simulink model "PC_Quadcopter_Simulation_Lyapnov_Hamilton"  (R2015b)
settings: Solver=FixedStepAuto  StartTime=0.0  StopTime=10  FixedStep=0.02  RelTol=1e-3
values from neighbouring files (symbols this model uses):
  IC = block.DialogPrm(2).Data    [QuadHamiSFunctionArticle.m]    (also in initialData.mat = )
  quadModel =     [initialData.mat]
undefined symbols (not defined in the file): K10, K11, K12, K7, K8, K9
settings Model: Creator=HKJ  LastModifiedBy=HL

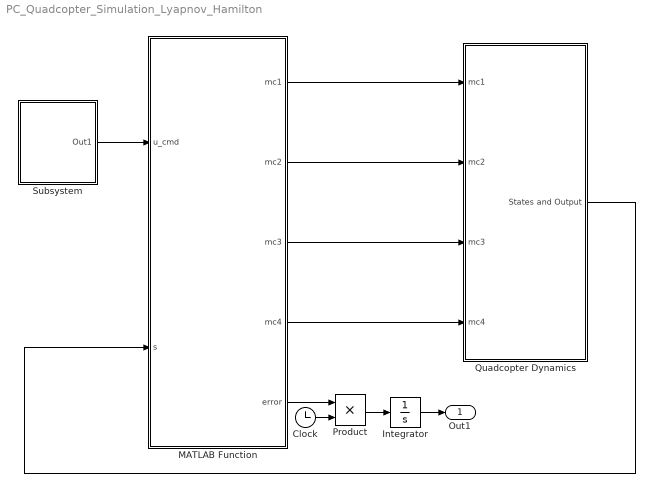
== system PC_Quadcopter_Simulation_Lyapnov_Hamilton ==
  Clock : Clock
  Integrator : Integrator
  MATLAB Function : MATLAB Function  TreatAsAtomicUnit=on  mask{k1=15, k2=8, k3=15, k4=8, k5=2.5, k6=2.5, k7=K7, k8=K8, k9=K9, k10=K10, k11=K11, k12=K12}
  Product : Product
  Quadcopter Dynamics : Subsystem
  Subsystem : Subsystem
  Out1 : Outport
  wires:
  MATLAB Function/1(mc1) -> Quadcopter Dynamics/1(mc1)
  MATLAB Function/2(mc2) -> Quadcopter Dynamics/2(mc2)
  MATLAB Function/3(mc3) -> Quadcopter Dynamics/3(mc3)
  MATLAB Function/4(mc4) -> Quadcopter Dynamics/4(mc4)
  Subsystem/1(Out1) -> MATLAB Function/1(u_cmd)
  Quadcopter Dynamics/1(States and Output) -> MATLAB Function/2(s)
  MATLAB Function/5(error) -> Product/1
  Clock/1 -> Product/2
  Product/1 -> Integrator/1
  Integrator/1 -> Out1/1

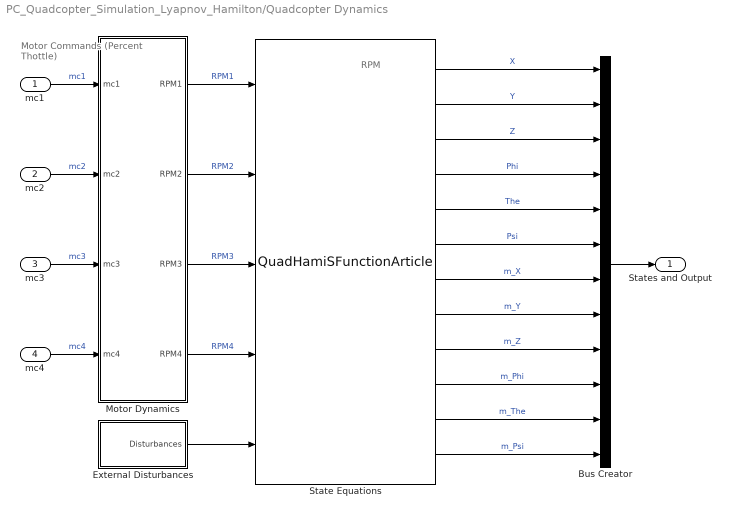
== system PC_Quadcopter_Simulation_Lyapnov_Hamilton/Quadcopter Dynamics ==
  note: Motor Commands
      | (Percent Thottle)
  note: RPM
  mc1 : Inport
  mc2 : Inport  Port=2
  mc3 : Inport  Port=3
  mc4 : Inport  Port=4
  Bus Creator : BusCreator  Inputs='X','Y','Z','Phi','The','Psi','m_X','m_Y','m_Z','m_Phi','m_The','m_Psi'
  External Disturbances : Subsystem
  Motor Dynamics : Subsystem
  State Equations : M-S-Function  FunctionName=QuadHamiSFunctionArticle  Parameters=quadModel,IC
      mask Display:
      | port_label('input', 1, 'RPM1')
      | port_label('input', 2, 'RPM2')
      | port_label('input', 3, 'RPM3')
      | port_label('input', 4, 'RPM4')
      | port_label('input', 5, 'Disturbances')
      | port_label('output', 1, 'X')
      | port_label('output', 2, 'Y')
      | port_label('output', 3, 'Z')
      | port_label('output', 4, 'Phi')
      | port_label('output', 5, 'The')
      | port_label('output', 6, 'Psi')
      | port_label('output', 7, 'm_X')
      | port_label('output', 8, 'm_Y')
      | port_label('output', 9, 'm_Z')
      | port_label('output', 10, 'm_Phi')
      | port_label('output', 11, 'm_The')
      | port_label('output', 12, 'm_Psi')
  States and Output : Outport
  wires:
  mc1/1 -> Motor Dynamics/1(mc1)  "mc1"
  mc2/1 -> Motor Dynamics/2(mc2)  "mc2"
  mc3/1 -> Motor Dynamics/3(mc3)  "mc3"
  mc4/1 -> Motor Dynamics/4(mc4)  "mc4"
  State Equations/1 -> Bus Creator/1  "X"
  State Equations/2 -> Bus Creator/2  "Y"
  State Equations/3 -> Bus Creator/3  "Z"
  State Equations/4 -> Bus Creator/4  "Phi"
  State Equations/5 -> Bus Creator/5  "The"
  State Equations/6 -> Bus Creator/6  "Psi"
  State Equations/7 -> Bus Creator/7  "m_X"
  State Equations/8 -> Bus Creator/8  "m_Y"
  State Equations/9 -> Bus Creator/9  "m_Z"
  State Equations/10 -> Bus Creator/10  "m_Phi"
  State Equations/11 -> Bus Creator/11  "m_The"
  State Equations/12 -> Bus Creator/12  "m_Psi"
  Bus Creator/1 -> States and Output/1
  Motor Dynamics/1(RPM1) -> State Equations/1  "RPM1"
  Motor Dynamics/2(RPM2) -> State Equations/2  "RPM2"
  Motor Dynamics/3(RPM3) -> State Equations/3  "RPM3"
  Motor Dynamics/4(RPM4) -> State Equations/4  "RPM4"
  External Disturbances/1("Disturbances ") -> State Equations/5

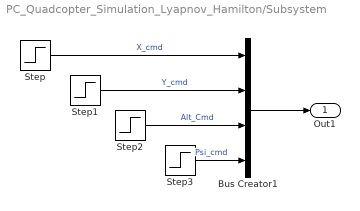
== system PC_Quadcopter_Simulation_Lyapnov_Hamilton/Subsystem ==
  Bus Creator1 : BusCreator  Inputs=4
  Step : Step  Time=0  SampleTime=0
  Step1 : Step  Time=0  SampleTime=0
  Step2 : Step  Time=0  After=-1  SampleTime=0
  Step3 : Step  Time=0  After=0  SampleTime=0
  Out1 : Outport
  wires:
  Step3/1 -> Bus Creator1/4  "Psi_cmd"
  Step2/1 -> Bus Creator1/3  "Alt_Cmd"
  Step/1 -> Bus Creator1/1  "X_cmd"
  Step1/1 -> Bus Creator1/2  "Y_cmd"
  Bus Creator1/1 -> Out1/1

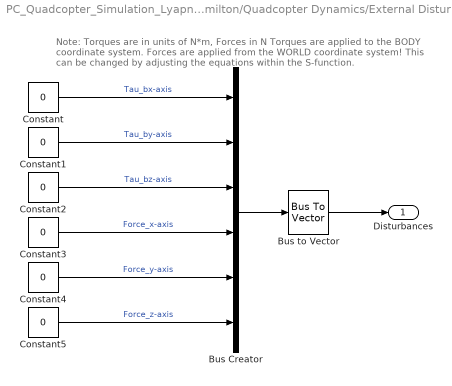
== system PC_Quadcopter_Simulation_Lyapnov_Hamilton/Quadcopter Dynamics/External Disturbances ==
  note: Note: Torques are in units of N*m, Forces in N
      | Torques are applied to the BODY coordinate system.
      | Forces are applied from the WORLD coordinate system!
      | This can be changed by adjusting the equations within the S-function.
  Bus Creator : BusCreator  Inputs=6
  Bus to Vector : BusToVector
  Constant{,1..5} (6 alike) : Constant  Value=0
  "Disturbances " : Outport
  wires:
  Bus to Vector/1 -> "Disturbances "/1
  Bus Creator/1 -> Bus to Vector/1
  Constant/1 -> Bus Creator/1  "Tau_bx-axis"
  Constant1/1 -> Bus Creator/2  "Tau_by-axis"
  Constant2/1 -> Bus Creator/3  "Tau_bz-axis"
  Constant3/1 -> Bus Creator/4  "Force_x-axis"
  Constant4/1 -> Bus Creator/5  "Force_y-axis"
  Constant5/1 -> Bus Creator/6  "Force_z-axis"

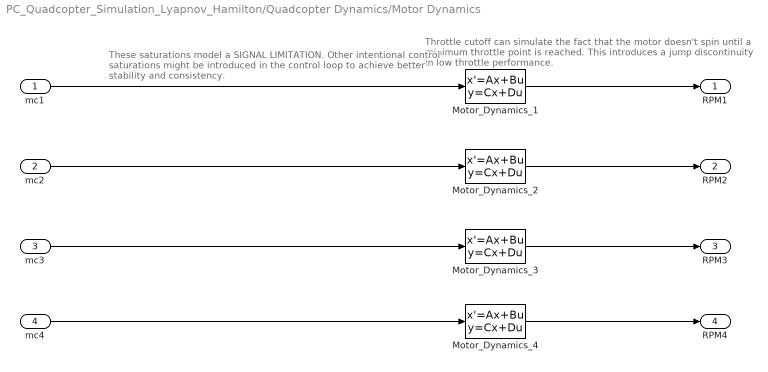
== system PC_Quadcopter_Simulation_Lyapnov_Hamilton/Quadcopter Dynamics/Motor Dynamics ==
  note: Throttle cutoff can simulate the fact that the motor doesn't
      | spin until a minimum throttle point is reached. This introduces
      | a jump discontinuity in low throttle performance.
  note: These saturations model a SIGNAL LIMITATION.
      | Other intentional control saturations might be introduced in the
      | control loop to achieve better stability and consistency.
  mc1 : Inport
  mc2 : Inport  Port=2
  mc3 : Inport  Port=3
  mc4 : Inport  Port=4
  Motor_Dynamics_1 : StateSpace  A=-1/quadModel.T  C=1/quadModel.T  D=0  X0=IC.w1*quadModel.T
  Motor_Dynamics_2 : StateSpace  A=-1/quadModel.T  C=1/quadModel.T  D=0  X0=IC.w2*quadModel.T
  Motor_Dynamics_3 : StateSpace  A=-1/quadModel.T  C=1/quadModel.T  D=0  X0=IC.w3*quadModel.T
  Motor_Dynamics_4 : StateSpace  A=-1/quadModel.T  C=1/quadModel.T  D=0  X0=IC.w4*quadModel.T
  RPM1 : Outport
  RPM2 : Outport  Port=2
  RPM3 : Outport  Port=3
  RPM4 : Outport  Port=4
  wires:
  mc1/1 -> Motor_Dynamics_1/1
  mc2/1 -> Motor_Dynamics_2/1
  mc3/1 -> Motor_Dynamics_3/1
  mc4/1 -> Motor_Dynamics_4/1
  Motor_Dynamics_1/1 -> RPM1/1
  Motor_Dynamics_2/1 -> RPM2/1
  Motor_Dynamics_3/1 -> RPM3/1
  Motor_Dynamics_4/1 -> RPM4/1

== matlab function PC_Quadcopter_Simulation_Lyapnov_Hamilton/MATLAB Function ==
  data: u_cmd input; mc1 output; s input; mc2 output; mc3 output; mc4 output; error output; k1 parameter; k2 parameter; k3 parameter; k4 parameter; k5 parameter; k6 parameter; k7 parameter; k8 parameter; k9 parameter; k10 parameter; k11 parameter; k12 parameter
function [mc1,mc2,mc3,mc4,error] = fcn(u_cmd,s, k1, k2, k3, k4, k5, k6, k7, k8, k9, k10, k11, k12)
%自己设计的控制器
% k1 = 15;
% k2 = 8;
% k3 = 15;
% k4 = 8;
% k5 = 2.5;
% k6 = 2.5;
% k7= 2;
% k8= 2;
% k9 = 2;
% k10 = 2;
% k11 = 2;
% k12 = 2;
Ix = 0.0094999;Iy=0.0094999;Iz=0.018576;
I = [Ix,0,0;0,Iy,0;0,0,Iz];
m=1.023;g=9.81;
% L=0.185738;%z这个值有问题
ct=1.4865e-07;
cq=2.925e-09;
ctl = 3.30374625e-08;

x_cmd = u_cmd(1);
y_cmd = u_cmd(2);
alt_cmd = u_cmd(3);
psi_cmd = u_cmd(4);
x = s(1);y = s(2);z = s(3);
Phi = s(4);The = s(5);Psi = s(6);
m_x = s(7);m_y = s(8);m_z = s(9);
m_Phi = s(10);m_The = s(11);m_Psi = s(12);

dPhi = (Iy*Iz+(Ix-Iz)*Iy*sin(The)^2-(Iy-Iz)*Ix*sin(Phi)^2*sin(The)^2)*m_Phi/(Ix*Iy*Iz*cos(The)^2)+...
       (-(Iy-Iz)*cos(Phi)*sin(Phi)*sin(The)*m_The)/(Iy*Iz*cos(The))+...
       (Iy*cos(Phi)^2+Iz*sin(Phi)^2)*sin(The)*m_Psi/(Iy*Iz*cos(The)^2);
dThe = -(Iy-Iz)*cos(Phi)*sin(Phi)*sin(The)*m_Phi/(Iy*Iz*cos(The))+...
       (Iy*sin(Phi)^2+Iz*cos(Phi)^2)*m_The/(Iy*Iz)+...
       (-(Iy-Iz)*cos(Phi)*sin(Phi))*m_Psi/(Iy*Iz*cos(The));
dPsi = (Iy*cos(Phi)^2+Iz*sin(Phi)^2)*sin(The)*m_Phi/(Iy*Iz*cos(The)^2)+...
       (-(Iy-Iz)*cos(Phi)*sin(Phi))*m_The/(Iy*Iz*cos(The))+...
       (Iy*cos(Phi)^2+Iz*sin(Phi)^2)*m_Psi/(Iy*Iz*cos(The)^2);

g1 = (Iy*Iz+(Ix-Iz)*Iy*sin(The)^2-(Iy-Iz)*Ix*sin(Phi)^2*sin(The)^2)/(Ix*Iy*Iz*cos(The)^2);
g2 = (Iy*sin(Phi)^2+Iz*cos(Phi)^2)/(Iy*Iz);
g3 = (Iy*cos(Phi)^2+Iz*sin(Phi)^2)/(Iy*Iz*cos(The)^2);

g12 = -(Iy-Iz)*cos(Phi)*sin(Phi)*sin(The)/(Iy*Iz*cos(The));
g13 = (Iy*cos(Phi)^2+Iz*sin(Phi)^2)*sin(The)/(Iy*Iz*cos(The)^2);
g23 = -(Iy-Iz)*cos(Phi)*sin(Phi)/(Iy*Iz*cos(The));

J = [g1,g12,g13;g12,g2,g23;g13,g23,g3];

f1 = -(Iy-Iz)*(dThe^2*sin(Phi)*cos(Phi)-dThe*dPsi*cos(2*Phi)*cos(The)-dPsi^2*sin(Phi)*cos(Phi)*cos(The)^2);
f2 = (Ix-Iy*sin(Phi)^2-Iz*cos(Phi)^2)*dPsi^2*sin(The)*cos(The)-(Iy-Iz)*dThe*dPsi*sin(Phi)*cos(Phi)*sin(The)-dPhi*dPsi*Ix*cos(The);


e7 = x - x_cmd;
e8 = m_x/m + k7*e7;
e9 = y - y_cmd;
e10 = m_y/m + k9*e9;
e11 = z-alt_cmd;
e12 = m_z/m+k11*e11;

alpha1 = m*((k7^2-1)*e7-(k7+k8)*e8);
alpha2 = m*((k9^2-1)*e9-(k9+k10)*e10);
alpha3 = -m*g+m*((k11^2-1)*e11-(k11+k12)*e12);
beta1 = alpha1*cos(Psi) + alpha2*sin(Psi);
beta2 = -alpha1*sin(Psi) + alpha2*cos(Psi);
beta3 = alpha3;
the_cmd = atan(beta1/beta3);
phi_cmd = atan(-beta2*cos(the_cmd)/beta3);
u1 = beta3/(cos(phi_cmd)*cos(the_cmd));

e1 = Phi-phi_cmd;
e2 = m_Phi/Ix+k1*e1;
e3 = The-the_cmd;
e4 = m_The/Iy+k3*e3;
e5 = Psi-psi_cmd;
e6 = m_Psi/Iz+k5*e5;

K_eta = [k1,0,0;0,k3,0;0,0,k5];
K_peta = [k2,0,0;0,k4,0;0,0,k6];
e_eta = [e1;e3;e5];
e_peta = [e2;e4;e6];
tau_p=I*((K_eta*J*I*K_eta-J*I)*e_eta-(K_eta+K_peta)*J*I*e_peta)-[f1;f2;0];
u2 = tau_p(1);
u3 = tau_p(2);
u4 = tau_p(3);

mc1 = sqrt((-u1/ct+u4/cq)*0.25+u3/ctl*0.5);
mc2 = sqrt((-u1/ct-u4/cq)*0.25+u2/ctl*0.5);
mc3 = sqrt((-u1/ct+u4/cq)*0.25-u3/ctl*0.5);
mc4 = sqrt((-u1/ct-u4/cq)*0.25-u2/ctl*0.5);

error = e7^2+e8^2+e9^2+e10^2+e11^2+e12^2;
